simulink subsystem "Sensing"  (R2024a)
settings: Solver=VariableStepAuto  StartTime=0.0  StopTime=10.0  RelTol=1e-3
undefined symbols (not defined in the file): Joint1_B, Joint1_F, Joint2_B, Joint2_F, Joint3_B, Joint3_F, MCU_Ts, Motor1, Motor2, Motor3, Motor_Rotationals, Payload_base_frame, Phase1_Pos, Phase2_Pos, Phase3_Pos, Phase_Neg, Transmission1_Stage2, Transmission2_Stage2, Transmission3_Stage1, Transmission_Rotationals
libraries: sm_lib x2, fl_lib x1, nesl_utility x1
settings Model: DataDictionary=neck_mk3.sldd  EnableAccessToBaseWorkspace=off  Creator=upattacini  LastModifiedBy=upattacini
settings RTWCC: GPUComputeCapability=3.5

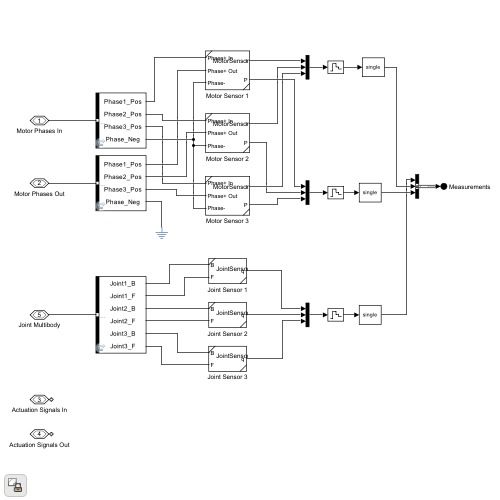
[thumbnail: Simulink's stored preview of the top-level diagram]
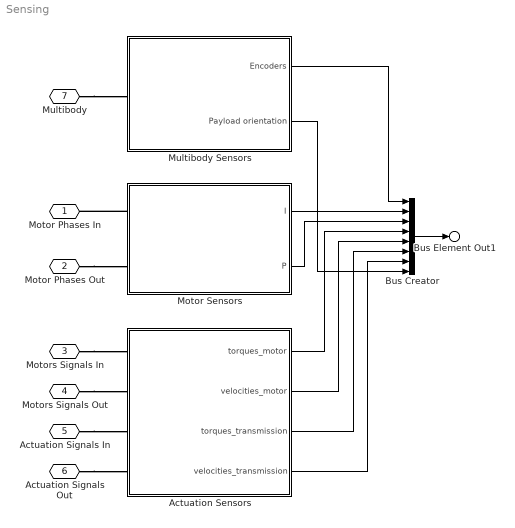
== system Sensing ==
  Actuation Sensors : Subsystem
      settings: PortSchema="{\"entries\":[{\"content\":{\"sides\":[{\"content\":{\"connectorIds\":[\"Out1\",\"Out2\",\"Out3\",\"Out4\"]},\"type\":\"ConnectorPlacement.EquallySpacedRectSide\",\"uuid\":\"610cdf94-cd3d-47b1-b3fb-2b07ba983e33\"},{\"content\":{\"connectorIds\":[\"RConn1\",\"RConn2\",\"RConn3\",\"RConn4\"],\"side\":\"RIGHT\"},\"type\":\"ConnectorPlacement.EquallySpacedRectSide\",\"uuid\":\"b6f9ab92-6c77-47ea-97aa-43f7fca8d359\"},{\"content\":{\"side\":\"TOP\"},\"type\":\"ConnectorPlacement.EquallySpacedRectSide\",\"uuid\":\"b6501941-3853-46ed-a483-71453a32dc77\"}]},\"type\":\"ConnectorPlacement.EquallySpacedConnector\",\"uuid\":\"510924d2-010e-4175-a97c-86b828b854ba\"}],\"packageUris\":[\"http://schema.mathworks.com/mf0/Connector/R2020b\"],\"version\":\"1.0\"}"
  Bus Creator : BusCreator  Inputs=8  OutDataTypeStr=Bus: Data_Measurements  NonVirtualBus=on
      settings: InheritFromInputs=off
  Motor Sensors : Subsystem
  Multibody Sensors : Subsystem
  Motor Phases In : PMIOPort  Side=Right  ConnectionType=Bus: Physical_MotorPhases
  Motor Phases Out : PMIOPort  Port=2  Side=Right  ConnectionType=Bus: Physical_MotorPhases
  Motors Signals In : PMIOPort  Port=3  Side=Right  ConnectionType=Bus: Physical_Actuation
  Motors Signals Out : PMIOPort  Port=4  Side=Right  ConnectionType=Bus: Physical_Actuation
  Actuation Signals In : PMIOPort  Port=5  Side=Right  ConnectionType=Bus: Physical_Actuation
  Actuation Signals Out : PMIOPort  Port=6  Side=Right  ConnectionType=Bus: Physical_Actuation
  Multibody : PMIOPort  Port=7  Side=Right  ConnectionType=Bus: Physical_Multibody
  Bus Element Out1 : Outport  PortName=Measurements
  wires:
  Bus Creator/1 -> Bus Element Out1/1
  Motor Sensors/1(I) -> Bus Creator/2
  Motor Sensors/2(P) -> Bus Creator/3
  Multibody Sensors/1(Encoders) -> Bus Creator/1
  Multibody Sensors/2(Payload orientation) -> Bus Creator/8
  Actuation Sensors/1(torques_motor) -> Bus Creator/4
  Actuation Sensors/2(velocities_motor) -> Bus Creator/5
  Actuation Sensors/3(torques_transmission) -> Bus Creator/6
  Actuation Sensors/4(velocities_transmission) -> Bus Creator/7
  connections:
  Actuation Signals Out/RConn1 -- Actuation Sensors/RConn4
  Motor Sensors/LConn1 -- Motor Phases In/RConn1
  Motor Phases Out/RConn1 -- Motor Sensors/LConn2
  Multibody/RConn1 -- Multibody Sensors/LConn1
  Actuation Signals In/RConn1 -- Actuation Sensors/RConn3
  Motors Signals In/RConn1 -- Actuation Sensors/RConn1
  Motors Signals Out/RConn1 -- Actuation Sensors/RConn2

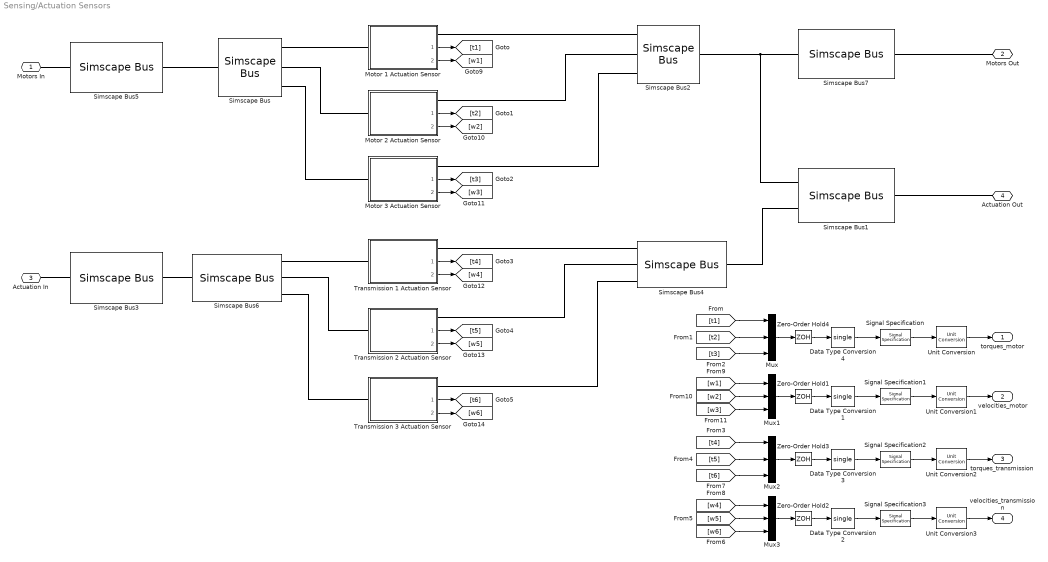
== system Sensing/Actuation Sensors ==
  Data Type Conversion{1..4} (4 alike) : DataTypeConversion  OutDataTypeStr=single  SaturateOnIntegerOverflow=off  RndMeth=Floor
  Motor 1 Actuation Sensor : Subsystem  ReferencedSubsystem=ActuationSensor
      settings: PortSchema="{\"entries\":[{\"content\":{\"sides\":[{\"content\":{\"connectorIds\":[\"LConn1\"]},\"type\":\"ConnectorPlacement.EquallySpacedRectSide\",\"uuid\":\"6301241c-4e88-40c2-a74e-d81256c12ae0\"},{\"content\":{\"connectorIds\":[\"RConn1\",\"Out1\",\"Out2\"],\"side\":\"RIGHT\"},\"type\":\"ConnectorPlacement.EquallySpacedRectSide\",\"uuid\":\"20e2936f-eff7-4744-b045-3c0d799baa7d\"},{\"content\":{\"side\":\"TOP\"},\"type\":\"ConnectorPlacement.EquallySpacedRectSide\",\"uuid\":\"551c152f-b5f1-40c6-80fe-f68509c5698c\"}]},\"type\":\"ConnectorPlacement.EquallySpacedConnector\",\"uuid\":\"41bd7279-be31-42ef-8e3a-e187726b4532\"}],\"packageUris\":[\"http://schema.mathworks.com/mf0/Connector/R2020b\"],\"version\":\"1.0\"}"
  Motor 2 Actuation Sensor : Subsystem  ReferencedSubsystem=ActuationSensor
      settings: PortSchema="{\"entries\":[{\"content\":{\"sides\":[{\"content\":{\"connectorIds\":[\"LConn1\"]},\"type\":\"ConnectorPlacement.EquallySpacedRectSide\",\"uuid\":\"6301241c-4e88-40c2-a74e-d81256c12ae0\"},{\"content\":{\"connectorIds\":[\"RConn1\",\"Out1\",\"Out2\"],\"side\":\"RIGHT\"},\"type\":\"ConnectorPlacement.EquallySpacedRectSide\",\"uuid\":\"20e2936f-eff7-4744-b045-3c0d799baa7d\"},{\"content\":{\"side\":\"TOP\"},\"type\":\"ConnectorPlacement.EquallySpacedRectSide\",\"uuid\":\"551c152f-b5f1-40c6-80fe-f68509c5698c\"}]},\"type\":\"ConnectorPlacement.EquallySpacedConnector\",\"uuid\":\"41bd7279-be31-42ef-8e3a-e187726b4532\"}],\"packageUris\":[\"http://schema.mathworks.com/mf0/Connector/R2020b\"],\"version\":\"1.0\"}"
  Motor 3 Actuation Sensor : Subsystem  ReferencedSubsystem=ActuationSensor
      settings: PortSchema="{\"entries\":[{\"content\":{\"sides\":[{\"content\":{\"connectorIds\":[\"LConn1\"]},\"type\":\"ConnectorPlacement.EquallySpacedRectSide\",\"uuid\":\"6301241c-4e88-40c2-a74e-d81256c12ae0\"},{\"content\":{\"connectorIds\":[\"RConn1\",\"Out1\",\"Out2\"],\"side\":\"RIGHT\"},\"type\":\"ConnectorPlacement.EquallySpacedRectSide\",\"uuid\":\"20e2936f-eff7-4744-b045-3c0d799baa7d\"},{\"content\":{\"side\":\"TOP\"},\"type\":\"ConnectorPlacement.EquallySpacedRectSide\",\"uuid\":\"551c152f-b5f1-40c6-80fe-f68509c5698c\"}]},\"type\":\"ConnectorPlacement.EquallySpacedConnector\",\"uuid\":\"41bd7279-be31-42ef-8e3a-e187726b4532\"}],\"packageUris\":[\"http://schema.mathworks.com/mf0/Connector/R2020b\"],\"version\":\"1.0\"}"
  Mux{,1..3} (4 alike) : Mux  Inputs=3
  Signal Specification : SignalSpecification  Unit=N*m
  Signal Specification1 : SignalSpecification  Unit=rad/s
  Signal Specification2 : SignalSpecification  Unit=N*m
  Signal Specification3 : SignalSpecification  Unit=rad/s
  Simscape Bus : SimscapeBus  HierarchyStrings=Motor1;Motor2;Motor3  ConnectionType=Bus: Physical_MotorRotationals
  Simscape Bus1 : SimscapeBus  HierarchyStrings=Motor_Rotationals;Transmission_Rotationals  ConnectionType=Bus: Physical_Actuation
  Simscape Bus2 : SimscapeBus  HierarchyStrings=Motor1;Motor2;Motor3  ConnectionType=Bus: Physical_MotorRotationals
  Simscape Bus3 : SimscapeBus  HierarchyStrings=Transmission_Rotationals  ConnectionType=Bus: Physical_Actuation
  Simscape Bus4 : SimscapeBus  HierarchyStrings=Transmission1_Stage2;Transmission2_Stage2;Transmission3_Stage1  ConnectionType=Bus: Physical_TransmissionRotationals
  Simscape Bus5 : SimscapeBus  HierarchyStrings=Motor_Rotationals  ConnectionType=Bus: Physical_Actuation
  Simscape Bus6 : SimscapeBus  HierarchyStrings=Transmission1_Stage2;Transmission2_Stage2;Transmission3_Stage1  ConnectionType=Bus: Physical_TransmissionRotationals
  Simscape Bus7 : SimscapeBus  HierarchyStrings=Motor_Rotationals  ConnectionType=Bus: Physical_Actuation
  Transmission 1 Actuation Sensor : Subsystem  ReferencedSubsystem=ActuationSensor
      settings: PortSchema="{\"entries\":[{\"content\":{\"sides\":[{\"content\":{\"connectorIds\":[\"LConn1\"]},\"type\":\"ConnectorPlacement.EquallySpacedRectSide\",\"uuid\":\"6301241c-4e88-40c2-a74e-d81256c12ae0\"},{\"content\":{\"connectorIds\":[\"RConn1\",\"Out1\",\"Out2\"],\"side\":\"RIGHT\"},\"type\":\"ConnectorPlacement.EquallySpacedRectSide\",\"uuid\":\"20e2936f-eff7-4744-b045-3c0d799baa7d\"},{\"content\":{\"side\":\"TOP\"},\"type\":\"ConnectorPlacement.EquallySpacedRectSide\",\"uuid\":\"551c152f-b5f1-40c6-80fe-f68509c5698c\"}]},\"type\":\"ConnectorPlacement.EquallySpacedConnector\",\"uuid\":\"41bd7279-be31-42ef-8e3a-e187726b4532\"}],\"packageUris\":[\"http://schema.mathworks.com/mf0/Connector/R2020b\"],\"version\":\"1.0\"}"
  Transmission 2 Actuation Sensor : Subsystem  ReferencedSubsystem=ActuationSensor
      settings: PortSchema="{\"entries\":[{\"content\":{\"sides\":[{\"content\":{\"connectorIds\":[\"LConn1\"]},\"type\":\"ConnectorPlacement.EquallySpacedRectSide\",\"uuid\":\"6301241c-4e88-40c2-a74e-d81256c12ae0\"},{\"content\":{\"connectorIds\":[\"RConn1\",\"Out1\",\"Out2\"],\"side\":\"RIGHT\"},\"type\":\"ConnectorPlacement.EquallySpacedRectSide\",\"uuid\":\"20e2936f-eff7-4744-b045-3c0d799baa7d\"},{\"content\":{\"side\":\"TOP\"},\"type\":\"ConnectorPlacement.EquallySpacedRectSide\",\"uuid\":\"551c152f-b5f1-40c6-80fe-f68509c5698c\"}]},\"type\":\"ConnectorPlacement.EquallySpacedConnector\",\"uuid\":\"41bd7279-be31-42ef-8e3a-e187726b4532\"}],\"packageUris\":[\"http://schema.mathworks.com/mf0/Connector/R2020b\"],\"version\":\"1.0\"}"
  Transmission 3 Actuation Sensor : Subsystem  ReferencedSubsystem=ActuationSensor
      settings: PortSchema="{\"entries\":[{\"content\":{\"sides\":[{\"content\":{\"connectorIds\":[\"LConn1\"]},\"type\":\"ConnectorPlacement.EquallySpacedRectSide\",\"uuid\":\"6301241c-4e88-40c2-a74e-d81256c12ae0\"},{\"content\":{\"connectorIds\":[\"RConn1\",\"Out1\",\"Out2\"],\"side\":\"RIGHT\"},\"type\":\"ConnectorPlacement.EquallySpacedRectSide\",\"uuid\":\"20e2936f-eff7-4744-b045-3c0d799baa7d\"},{\"content\":{\"side\":\"TOP\"},\"type\":\"ConnectorPlacement.EquallySpacedRectSide\",\"uuid\":\"551c152f-b5f1-40c6-80fe-f68509c5698c\"}]},\"type\":\"ConnectorPlacement.EquallySpacedConnector\",\"uuid\":\"41bd7279-be31-42ef-8e3a-e187726b4532\"}],\"packageUris\":[\"http://schema.mathworks.com/mf0/Connector/R2020b\"],\"version\":\"1.0\"}"
  Unit Conversion{,1..3} (4 alike) : UnitConversion
  Zero-Order Hold{1..4} (4 alike) : ZeroOrderHold  SampleTime=MCU_Ts
  Motors In : PMIOPort  Side=Right
  Motors Out : PMIOPort  Port=2  Side=Right
  Actuation In : PMIOPort  Port=3  Side=Right
  Actuation Out : PMIOPort  Port=4  Side=Right
  torques_motor : Outport
  velocities_motor : Outport  Port=2
  torques_transmission : Outport  Port=3
  velocities_transmission : Outport  Port=4
  wires:
  Signal Specification3/1 -> Unit Conversion3/1
  Signal Specification2/1 -> Unit Conversion2/1
  Unit Conversion3/1 -> velocities_transmission/1
  Unit Conversion2/1 -> torques_transmission/1
  Unit Conversion1/1 -> velocities_motor/1
  Data Type Conversion1/1 -> Signal Specification1/1
  Signal Specification1/1 -> Unit Conversion1/1
  Signal Specification/1 -> Unit Conversion/1
  Unit Conversion/1 -> torques_motor/1
  Mux3/1 -> Zero-Order Hold2/1
  Mux2/1 -> Zero-Order Hold3/1
  Mux1/1 -> Zero-Order Hold1/1
  Mux/1 -> Zero-Order Hold4/1
  [t4] -> Mux2/1
  [t5] -> Mux2/2
  [t6] -> Mux2/3
  [w6] -> Mux3/3
  [w5] -> Mux3/2
  [w4] -> Mux3/1
  Zero-Order Hold3/1 -> Data Type Conversion3/1
  Data Type Conversion3/1 -> Signal Specification2/1
  Zero-Order Hold2/1 -> Data Type Conversion2/1
  Data Type Conversion2/1 -> Signal Specification3/1
  Zero-Order Hold1/1 -> Data Type Conversion1/1
  Data Type Conversion4/1 -> Signal Specification/1
  Zero-Order Hold4/1 -> Data Type Conversion4/1
  Transmission 3 Actuation Sensor/2 -> [w6]
  Transmission 3 Actuation Sensor/1 -> [t6]
  Transmission 2 Actuation Sensor/2 -> [w5]
  Transmission 2 Actuation Sensor/1 -> [t5]
  Transmission 1 Actuation Sensor/2 -> [w4]
  Transmission 1 Actuation Sensor/1 -> [t4]
  Motor 3 Actuation Sensor/2 -> [w3]
  Motor 3 Actuation Sensor/1 -> [t3]
  Motor 2 Actuation Sensor/2 -> [w2]
  Motor 2 Actuation Sensor/1 -> [t2]
  [w1] -> Mux1/1
  [w2] -> Mux1/2
  [w3] -> Mux1/3
  [t3] -> Mux/3
  [t2] -> Mux/2
  [t1] -> Mux/1
  Motor 1 Actuation Sensor/2 -> [w1]
  Motor 1 Actuation Sensor/1 -> [t1]
  connections:
  Motors Out/RConn1 -- Simscape Bus7/RConn1
  Simscape Bus1/LConn1 -- Simscape Bus2/RConn1 -- Simscape Bus7/LConn1
  Simscape Bus5/LConn1 -- Simscape Bus/RConn1
  Motors In/RConn1 -- Simscape Bus5/RConn1
  Simscape Bus4/LConn3 -- Transmission 3 Actuation Sensor/RConn1
  Simscape Bus4/LConn2 -- Transmission 2 Actuation Sensor/RConn1
  Simscape Bus6/LConn3 -- Transmission 3 Actuation Sensor/LConn1
  Simscape Bus6/LConn2 -- Transmission 2 Actuation Sensor/LConn1
  Simscape Bus4/LConn1 -- Transmission 1 Actuation Sensor/RConn1
  Simscape Bus6/LConn1 -- Transmission 1 Actuation Sensor/LConn1
  Motor 3 Actuation Sensor/RConn1 -- Simscape Bus2/LConn3
  Motor 2 Actuation Sensor/RConn1 -- Simscape Bus2/LConn2
  Simscape Bus6/RConn1 -- Simscape Bus3/LConn1
  Simscape Bus4/RConn1 -- Simscape Bus1/LConn2
  Motor 1 Actuation Sensor/RConn1 -- Simscape Bus2/LConn1
  Simscape Bus1/RConn1 -- Actuation Out/RConn1
  Motor 3 Actuation Sensor/LConn1 -- Simscape Bus/LConn3
  Motor 2 Actuation Sensor/LConn1 -- Simscape Bus/LConn2
  Simscape Bus/LConn1 -- Motor 1 Actuation Sensor/LConn1
  Simscape Bus3/RConn1 -- Actuation In/RConn1

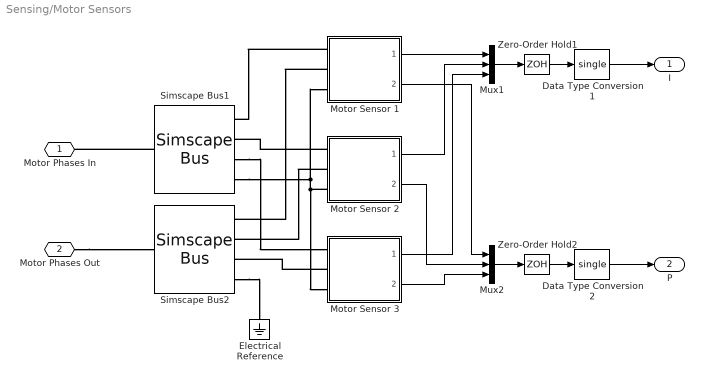
== system Sensing/Motor Sensors ==
  Data Type Conversion1 : DataTypeConversion  OutDataTypeStr=single  SaturateOnIntegerOverflow=off  RndMeth=Floor
  Data Type Conversion2 : DataTypeConversion  OutDataTypeStr=single  SaturateOnIntegerOverflow=off  RndMeth=Floor
  Electrical Reference : fl_lib/Electrical/Electrical Elements/Electrical Reference
  Motor Sensor 1 : Subsystem  ReferencedSubsystem=MotorSensor
  Motor Sensor 2 : Subsystem  ReferencedSubsystem=MotorSensor
  Motor Sensor 3 : Subsystem  ReferencedSubsystem=MotorSensor
  Mux1 : Mux  Inputs=3
  Mux2 : Mux  Inputs=3
  Simscape Bus1 : SimscapeBus  HierarchyStrings=Phase1_Pos;Phase2_Pos;Phase3_Pos;Phase_Neg  ConnectionType=Bus: Physical_MotorPhases
  Simscape Bus2 : SimscapeBus  HierarchyStrings=Phase1_Pos;Phase2_Pos;Phase3_Pos;Phase_Neg  ConnectionType=Bus: Physical_MotorPhases
  Zero-Order Hold1 : ZeroOrderHold  SampleTime=MCU_Ts
  Zero-Order Hold2 : ZeroOrderHold  SampleTime=MCU_Ts
  Motor Phases In : PMIOPort  Side=Left
  Motor Phases Out : PMIOPort  Port=2  Side=Left
  I : Outport
  P : Outport  Port=2
  wires:
  Data Type Conversion2/1 -> P/1
  Data Type Conversion1/1 -> I/1
  Mux2/1 -> Zero-Order Hold2/1
  Mux1/1 -> Zero-Order Hold1/1
  Zero-Order Hold2/1 -> Data Type Conversion2/1
  Zero-Order Hold1/1 -> Data Type Conversion1/1
  Motor Sensor 2/1 -> Mux1/2
  Motor Sensor 3/2 -> Mux2/3
  Motor Sensor 2/2 -> Mux2/2
  Motor Sensor 1/1 -> Mux1/1
  Motor Sensor 3/1 -> Mux1/3
  Motor Sensor 1/2 -> Mux2/1
  connections:
  Motor Phases Out/RConn1 -- Simscape Bus2/RConn1
  Simscape Bus1/LConn3 -- Motor Sensor 3/LConn1
  Motor Sensor 1/LConn1 -- Simscape Bus1/LConn1
  Simscape Bus1/RConn1 -- Motor Phases In/RConn1
  Motor Sensor 2/LConn1 -- Simscape Bus1/LConn2
  Motor Sensor 1/LConn2 -- Simscape Bus2/LConn1
  Simscape Bus2/LConn4 -- Electrical Reference/LConn1
  Motor Sensor 3/LConn2 -- Simscape Bus2/LConn3
  Motor Sensor 2/LConn3 -- Motor Sensor 3/LConn3 -- Simscape Bus1/LConn4 -- Motor Sensor 1/LConn3
  Motor Sensor 2/LConn2 -- Simscape Bus2/LConn2

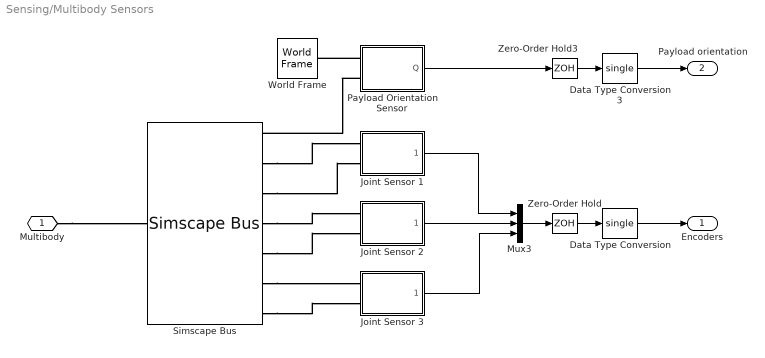
== system Sensing/Multibody Sensors ==
  Data Type Conversion : DataTypeConversion  OutDataTypeStr=single  SaturateOnIntegerOverflow=off  RndMeth=Floor
  Data Type Conversion3 : DataTypeConversion  OutDataTypeStr=single  SaturateOnIntegerOverflow=off  RndMeth=Floor
  Joint Sensor 1 : Subsystem  ReferencedSubsystem=JointSensor
  Joint Sensor 2 : Subsystem  ReferencedSubsystem=JointSensor
  Joint Sensor 3 : Subsystem  ReferencedSubsystem=JointSensor
  Mux3 : Mux  Inputs=3
  Payload Orientation Sensor : Subsystem
  Simscape Bus : SimscapeBus  HierarchyStrings=Payload_base_frame;Joint1_B;Joint1_F;Joint2_B;Joint2_F;Joint3_B;Joint3_F  ConnectionType=Bus: Physical_Multibody
  World Frame : sm_lib/Frames and Transforms/World Frame
  Zero-Order Hold : ZeroOrderHold  SampleTime=MCU_Ts
  Zero-Order Hold3 : ZeroOrderHold  SampleTime=MCU_Ts
  Multibody : PMIOPort  Side=Left
  Encoders : Outport
  Payload orientation : Outport  Port=2
  wires:
  Data Type Conversion3/1 -> Payload orientation/1
  Data Type Conversion/1 -> Encoders/1
  Zero-Order Hold/1 -> Data Type Conversion/1
  Joint Sensor 2/1 -> Mux3/2
  Joint Sensor 1/1 -> Mux3/1
  Mux3/1 -> Zero-Order Hold/1
  Joint Sensor 3/1 -> Mux3/3
  Payload Orientation Sensor/1(Q) -> Zero-Order Hold3/1
  Zero-Order Hold3/1 -> Data Type Conversion3/1
  connections:
  Simscape Bus/LConn6 -- Joint Sensor 3/LConn1
  Simscape Bus/LConn5 -- Joint Sensor 2/LConn2
  Payload Orientation Sensor/LConn1 -- World Frame/RConn1
  Payload Orientation Sensor/LConn2 -- Simscape Bus/LConn1
  Simscape Bus/LConn2 -- Joint Sensor 1/LConn1
  Simscape Bus/LConn4 -- Joint Sensor 2/LConn1
  Simscape Bus/LConn3 -- Joint Sensor 1/LConn2
  Multibody/RConn1 -- Simscape Bus/RConn1
  Simscape Bus/LConn7 -- Joint Sensor 3/LConn2

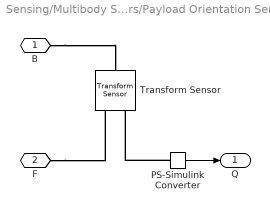
== system Sensing/Multibody Sensors/Payload Orientation Sensor ==
  PS-Simulink Converter : nesl_utility/PS-Simulink Converter  PhysicalDomain=network_engine_domain  SubClassName=ps_output  LeftPortType=input  RightPortType=output  PseudoPeriodic=off  Frequencies=[]  VectorFormat=inherit  Unit=1  AffineConversion=off
  Transform Sensor : sm_lib/Frames and Transforms/Transform Sensor  MeasurementFrame=Base  RotationSequence=XYX  SenseAngle=off  SenseAxis=off  SenseQ=on  SenseR=off  SenseRotationSequence=off  SenseOmegaX=off  SenseOmegaY=off  SenseOmegaZ=off  SenseOmega=off  SenseQDot=off  SenseRDot=off  SenseRotationSequenceDot=off  SenseAlphaX=off  SenseAlphaY=off  SenseAlphaZ=off  SenseAlpha=off  SenseQDDot=off  SenseRDDot=off  SenseX=off  SenseY=off  SenseZ=off  SenseXYZ=off  SenseRad=off  SenseAzim=off  SenseDist=off  SenseInc=off  SenseXDot=off  SenseYDot=off  SenseZDot=off  SenseXYZDot=off  SenseRadDot=off  SenseAzimDot=off  SenseDistDot=off  SenseIncDot=off  SenseXDDot=off  SenseYDDot=off  SenseZDDot=off  SenseXYZDDot=off  SenseRadDDot=off  SenseAzimDDot=off  SenseDistDDot=off  SenseIncDDot=off
  B : PMIOPort  Side=Left
  F : PMIOPort  Port=2  Side=Left
  Q : Outport
  wires:
  PS-Simulink Converter/1 -> Q/1
  connections:
  PS-Simulink Converter/LConn1 -- Transform Sensor/RConn2
  B/RConn1 -- Transform Sensor/LConn1
  F/RConn1 -- Transform Sensor/RConn1
